simulink model "model"  (R2019b)
settings: Solver=VariableStepAuto  StartTime=0.0  StopTime=20.0  RelTol=1e-3
values from neighbouring files (symbols this model uses):
  A_down = [0 0 1 0;0 0 0 1;0 52.8369133 -19.50692833 0.6541334519;0 -98.08151611 19.46859916 -1.214272309]    [Lab.m]
  B_down = 2.6*[0;0;35.06604733;-34.99714604]    [Lab.m]
  K_down_LQR = lqr(A_down, B_down, Q_down, R_down)    [Lab.m]
  K_up = acker(A_up, B_up, P2)    [Lab.m]
  K_up_LQR = lqr(A_up, B_up, Q_up, R_up)    [Lab.m]
libraries: simulink_extras x2
settings Model: Creator=miaokeyan  LastModifiedBy=miaokeyan

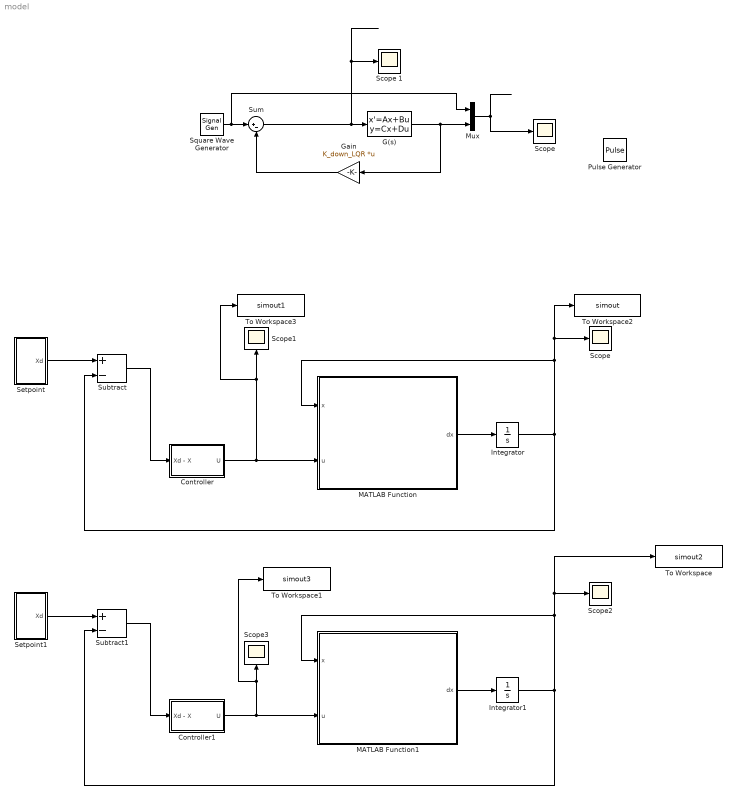
== system model ==
  Controller : Subsystem
  Controller1 : Subsystem
  G(s) : StateSpace  A=A_down  B=B_down  C=[1 0 0 0;0 1 0 0; 0 0 1 0; 0 0 0 1]  D=[0;0;0;0]  InitialCondition=0
  Gain : Gain  Gain=K_down_LQR  Multiplication=Matrix(K*u) (u vector)
  Integrator : Integrator  InitialCondition=[0 0.1 0.1 0]
  Integrator1 : Integrator  InitialCondition=[0 0.1 0.1 0]
  MATLAB Function : MATLAB Function  TreatAsAtomicUnit=on
  MATLAB Function1 : MATLAB Function  TreatAsAtomicUnit=on
  Mux : Mux  Inputs=2
  Pulse Generator : DiscretePulseGenerator  PulseType=Time based  Period=10  PulseWidth=5
  Scope{,1..3} (4 alike) : Scope
  "Scope " : Scope
  Scope 1 : Scope
  Setpoint : Subsystem
  Setpoint1 : Subsystem
  Square Wave Generator : SignalGenerator  WaveForm=square  Frequency=0.2
  Subtract : Sum  Inputs=+-
  Subtract1 : Sum  Inputs=+-
  Sum : Sum  Inputs=|+-
  To Workspace : ToWorkspace  VariableName=simout2  SaveFormat=Timeseries  SampleTime=-1
  To Workspace1 : ToWorkspace  VariableName=simout3  SaveFormat=Timeseries  SampleTime=-1
  To Workspace2 : ToWorkspace  VariableName=simout  SaveFormat=Timeseries  SampleTime=-1
  To Workspace3 : ToWorkspace  VariableName=simout1  SaveFormat=Timeseries  SampleTime=-1
  wires:
  Mux/1 -> "Scope "/1
  Gain/1 -> Sum/2
  G(s)/1 -> Mux/2, Gain/1
  Sum/1 -> Scope 1/1, G(s)/1
  Square Wave Generator/1 -> Mux/1, Sum/1
  MATLAB Function/1(dx) -> Integrator/1
  Integrator/1 -> To Workspace2/1, Scope/1, MATLAB Function/1(x), Subtract/2
  Setpoint/1(Xd) -> Subtract/1
  Subtract/1 -> Controller/1(Xd - X)
  Controller/1(U) -> MATLAB Function/2(u), To Workspace3/1, Scope1/1
  Integrator1/1 -> To Workspace/1, Scope2/1, MATLAB Function1/1(x), Subtract1/2
  Controller1/1(U) -> MATLAB Function1/2(u), Scope3/1, To Workspace1/1
  Setpoint1/1(Xd) -> Subtract1/1
  Subtract1/1 -> Controller1/1(Xd - X)
  MATLAB Function1/1(dx) -> Integrator1/1

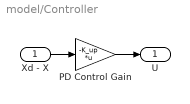
== system model/Controller ==
  Xd - X : Inport
  PD Control Gain : Gain  Gain=-K_up  Multiplication=Matrix(K*u)
  U : Outport
  wires:
  Xd - X/1 -> PD Control Gain/1
  PD Control Gain/1 -> U/1

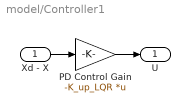
== system model/Controller1 ==
  Xd - X : Inport
  PD Control Gain : Gain  Gain=-K_up_LQR  Multiplication=Matrix(K*u)
  U : Outport
  wires:
  Xd - X/1 -> PD Control Gain/1
  PD Control Gain/1 -> U/1

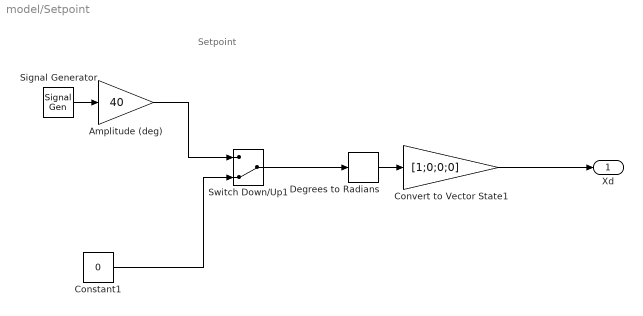
== system model/Setpoint ==
  note: Setpoint
  Amplitude (deg) : Gain  Gain=40  SaturateOnIntegerOverflow=on  OutDataTypeStr=Inherit: Same as input  ParamDataTypeStr=Inherit: Same as input
  Constant1 : Constant  Value=0
  Convert to Vector State1 : Gain  Gain=[1;0;0;0]
  Degrees to Radians : simulink_extras/Transformations/Degrees to Radians
  Signal Generator : SignalGenerator  WaveForm=square  Frequency=0.2
  Switch Down/Up1 : ManualSwitch  CurrentSetting=0
  Xd : Outport
  wires:
  Degrees to Radians/1 -> Convert to Vector State1/1
  Convert to Vector State1/1 -> Xd/1
  Signal Generator/1 -> Amplitude (deg)/1
  Constant1/1 -> Switch Down/Up1/2
  Amplitude (deg)/1 -> Switch Down/Up1/1
  Switch Down/Up1/1 -> Degrees to Radians/1

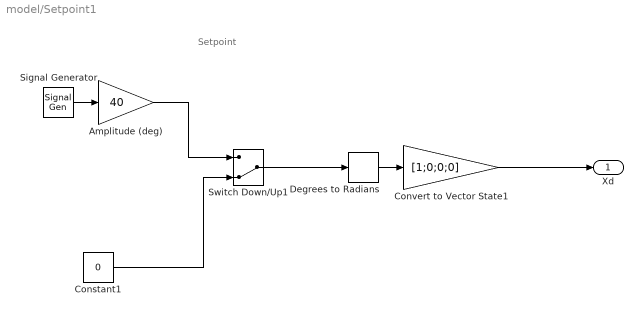
== system model/Setpoint1 ==
  note: Setpoint
  Amplitude (deg) : Gain  Gain=40  SaturateOnIntegerOverflow=on  OutDataTypeStr=Inherit: Same as input  ParamDataTypeStr=Inherit: Same as input
  Constant1 : Constant  Value=0
  Convert to Vector State1 : Gain  Gain=[1;0;0;0]
  Degrees to Radians : simulink_extras/Transformations/Degrees to Radians
  Signal Generator : SignalGenerator  WaveForm=square  Frequency=0.2
  Switch Down/Up1 : ManualSwitch  CurrentSetting=0
  Xd : Outport
  wires:
  Degrees to Radians/1 -> Convert to Vector State1/1
  Convert to Vector State1/1 -> Xd/1
  Signal Generator/1 -> Amplitude (deg)/1
  Constant1/1 -> Switch Down/Up1/2
  Amplitude (deg)/1 -> Switch Down/Up1/1
  Switch Down/Up1/1 -> Degrees to Radians/1

== matlab function model/MATLAB Function1 ==
  data: x input; dx output; u input
function dx = fcn(x,u)
% F = 1;
% M = 1;
% L = 0.842;
% g = 9.8093;
% dx = zeros(4,1);
% % K = [103.0043  112.5880  687.6229  137.7411];
% % u = K * [x1; x2; x3; x4];
A_up = [0,0,1,0;0,0,0,1;0,52.8369133000000,-19.5069283300000,-0.654133451900000;0,98.0815161100000,-19.4685991600000,-1.21427230900000];
B_up = [0;0;91.1717230580000;90.9925797040000];
dx = A_up * x - B_up * u;

== matlab function model/MATLAB Function ==
  data: x input; dx output; u input
function dx = fcn(x,u)
% F = 1;
% M = 1;
% L = 0.842;
% g = 9.8093;
% dx = zeros(4,1);
% % K = [103.0043  112.5880  687.6229  137.7411];
% % u = K * [x1; x2; x3; x4];
A_up = [0,0,1,0;0,0,0,1;0,52.8369133000000,-19.5069283300000,-0.654133451900000;0,98.0815161100000,-19.4685991600000,-1.21427230900000];
B_up = [0;0;91.1717230580000;90.9925797040000];
dx = A_up * x - B_up * u;
